simulink model "Book6242"  (R2019b)
settings: Solver=ode45  StartTime=0.0  StopTime=40  FixedStep=0.001  RelTol=1e-3
libraries: fuzblock x2
settings Model: Creator=user  LastModifiedBy=xyh

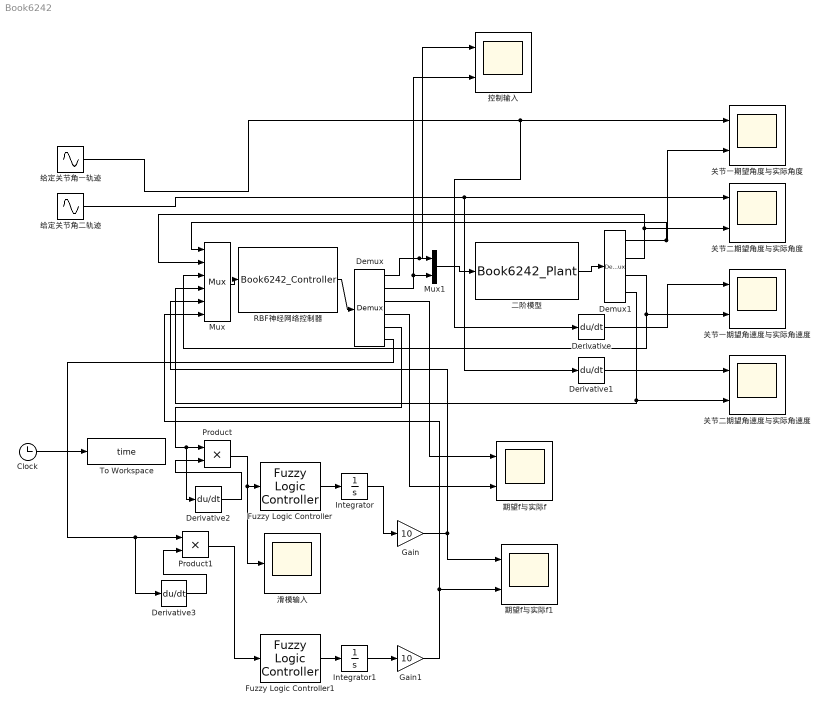
== system Book6242 ==
  Clock : Clock
  Demux : Demux  Outputs=6
  Demux1 : Demux
  Derivative{,1..3} (4 alike) : Derivative
  Fuzzy Logic Controller : fuzblock/Fuzzy Logic  Controller  FIS=Book6242  OutputSampleNumber=101  DataType=double  FuzzifiedInputs=off  RuleFiringStrengths=off  RuleOutputs=off  AggregatedOutputs=off  SimulateUsing=Interpreted execution  OutOfRangeInputValueMessage=warning  NoRuleFiredMessage=warning  EmptyOutputFuzzySetMessage=warning
  Fuzzy Logic Controller1 : fuzblock/Fuzzy Logic  Controller  FIS=Book6242  OutputSampleNumber=101  DataType=double  FuzzifiedInputs=off  RuleFiringStrengths=off  RuleOutputs=off  AggregatedOutputs=off  SimulateUsing=Interpreted execution  OutOfRangeInputValueMessage=warning  NoRuleFiredMessage=warning  EmptyOutputFuzzySetMessage=warning
  Gain : Gain  Gain=10
  Gain1 : Gain  Gain=10
  Integrator : Integrator
  Integrator1 : Integrator
  Mux : Mux  Inputs=6
  Mux1 : Mux  Inputs=2
  Product : Product
  Product1 : Product
  RBF神经网络控制器 : S-Function  FunctionName=Book6242_Controller  SFunctionDeploymentMode=off  EnableBusSupport=off
  To Workspace : ToWorkspace  VariableName=time  SaveFormat=Timeseries  SampleTime=-1
  二阶模型 : S-Function  FunctionName=Book6242_Plant  SFunctionDeploymentMode=off  EnableBusSupport=off
  关节一期望角度与实际角度 : Scope  NumInputPorts=2
  关节一期望角速度与实际角速度 : Scope  NumInputPorts=2
  关节二期望角度与实际角度 : Scope  NumInputPorts=2
  关节二期望角速度与实际角速度 : Scope  NumInputPorts=2
  控制输入 : Scope  NumInputPorts=2
  期望f与实际f : Scope  NumInputPorts=2
  期望f与实际f1 : Scope  NumInputPorts=2
  滑模输入 : Scope
  给定关节角一轨迹 : Sin  Amplitude=0.1  SampleTime=0
  给定关节角二轨迹 : Sin  Amplitude=0.1  SampleTime=0
  wires:
  Mux/1 -> RBF神经网络控制器/1
  Demux1/4 -> Mux/4, 关节二期望角速度与实际角速度/2
  Derivative1/1 -> 关节二期望角速度与实际角速度/1
  Demux/4 -> 期望f与实际f/2
  给定关节角一轨迹/1 -> Derivative/1, 关节一期望角度与实际角度/1
  Demux1/2 -> Mux/2, 关节二期望角度与实际角度/2
  RBF神经网络控制器/1 -> Demux/1
  Demux1/3 -> Mux/3, 关节一期望角速度与实际角速度/2
  Mux1/1 -> 二阶模型/1
  Demux1/1 -> Mux/1, 关节一期望角度与实际角度/2
  Demux/2 -> 控制输入/2, Mux1/2
  Demux/1 -> 控制输入/1, Mux1/1
  给定关节角二轨迹/1 -> 关节二期望角度与实际角度/1, Derivative1/1
  Derivative/1 -> 关节一期望角速度与实际角速度/1
  Clock/1 -> To Workspace/1
  二阶模型/1 -> Demux1/1
  Demux/3 -> 期望f与实际f/1
  Demux/6 -> Derivative3/1, Product1/1
  Demux/5 -> Derivative2/1, Product/1
  Fuzzy Logic Controller/1 -> Integrator/1
  Integrator/1 -> Gain/1
  Gain/1 -> Mux/5, 期望f与实际f1/1
  Integrator1/1 -> Gain1/1
  Fuzzy Logic Controller1/1 -> Integrator1/1
  Gain1/1 -> 期望f与实际f1/2, Mux/6
  Derivative2/1 -> Product/2
  Product/1 -> 滑模输入/1, Fuzzy Logic Controller/1
  Derivative3/1 -> Product1/2
  Product1/1 -> Fuzzy Logic Controller1/1
